simulink model "m_seg_var_simulink"  (R2022a)
settings: Solver=FixedStepAuto  StartTime=0.0  StopTime=60  FixedStep=0.01  RelTol=1e-3
values from neighbouring files (symbols this model uses):
  A = importdata('matrix_A1lin.txt')    [TestePID.m]    (also in lqrdovini.m; m_aloc.m; m_aloc2.m; m_lqr.m)
  B2 = B    [m_seg_cte.m]    (also in m_seg_var.m = importdata('matrix_B1lin.txt'); m_seg_var_main_simulink.m = importdata('matrix_B1lin.txt'); observador_aloc.m = importdata('matrix_B1lin.txt'); observador_lqr.m = importdata('matrix_B1lin.txt'))
  C = importdata('matrix_C1.txt')    [TestePID.m]    (also in lqrdovini.m; m_aloc.m; m_aloc2.m; m_lqr.m)
  D = importdata('matrix_D1.txt')    [TestePID.m]    (also in lqrdovini.m; m_aloc.m; m_aloc2.m; m_lqr.m)
  K = lqr(A,B,Q,P)    [lqrdovini.m]    (also in m_aloc.m = place(A,B,p); m_aloc2.m = place(A,B,p); m_lqr.m; m_seg_cte.m = place(A,B,p))
  Nu = N(7:9,:)    [m_seg_cte.m]    (also in m_seg_var_main_simulink.m)
  Nx = N(1:6,:)    [m_seg_cte.m]    (also in m_seg_var_main_simulink.m)
  xq_r = [q_r(2:4),x_r(4:6)]    [m_seg_var.m]    (also in m_seg_var_main_simulink.m; ref_var.m; teste_var.m)
settings Model: Creator=gusta  LastModifiedBy=gusta

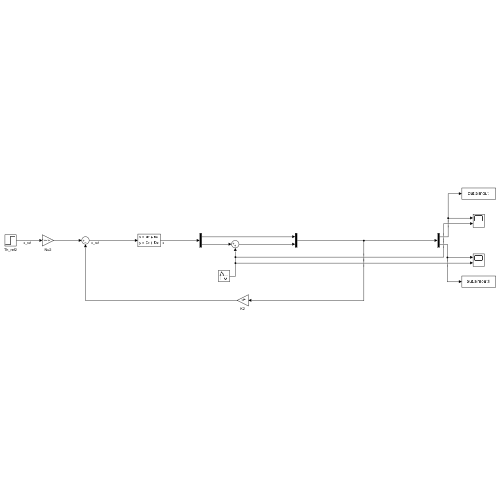
[thumbnail: Simulink's stored preview of the top-level diagram]
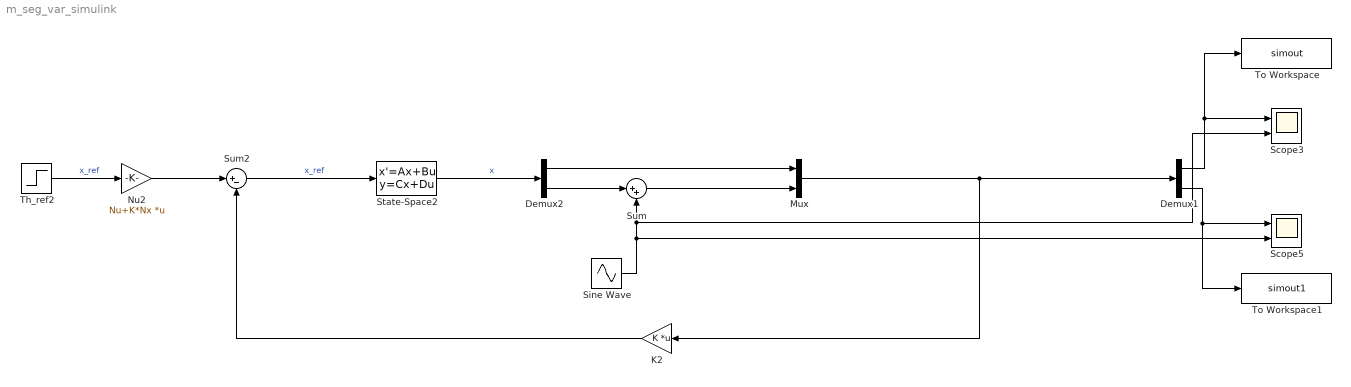
== system m_seg_var_simulink ==
  Demux1 : Demux  Outputs=2
  Demux2 : Demux  Outputs=2
  K2 : Gain  Gain=K  Multiplication=Matrix(K*u)
  Mux : Mux  Inputs=2
  Nu2 : Gain  Gain=Nu+K*Nx  Multiplication=Matrix(K*u) (u vector)
  Scope3 : Scope  NumInputPorts=2
  Scope5 : Scope  NumInputPorts=2
  Sine Wave : Sin  Amplitude=0.02  Frequency=0.5  SampleTime=0
  State-Space2 : StateSpace  A=A  B=B2  C=C  D=D  InitialCondition=0
  Sum : Sum  Inputs=|++
  Sum2 : Sum  Inputs=|+-
  Th_ref2 : Step  Time=0  After=xq_r*0  SampleTime=0  VectorParams1D=off
  To Workspace : ToWorkspace  VariableName=simout  SaveFormat=Timeseries  SampleTime=-1
  To Workspace1 : ToWorkspace  VariableName=simout1  SaveFormat=Timeseries  SampleTime=-1
  wires:
  Demux1/2 -> To Workspace1/1, Scope5/1
  Demux1/1 -> To Workspace/1, Scope3/1
  K2/1 -> Sum2/2
  Th_ref2/1 -> Nu2/1  "x_ref"
  Nu2/1 -> Sum2/1
  Sum2/1 -> State-Space2/1  "x_ref"
  Sine Wave/1 -> Scope5/2, Scope3/2, Sum/2
  State-Space2/1 -> Demux2/1  "x"
  Mux/1 -> K2/1, Demux1/1
  Demux2/1 -> Mux/1
  Demux2/2 -> Sum/1
  Sum/1 -> Mux/2
